simulink model "PolyMIMOsystem"  (R2021b)
settings: Solver=VariableStepAuto  StartTime=0.0  StopTime=Nsim  RelTol=1e-3
values from neighbouring files (symbols this model uses):
  myseed = [7; 27]    [dataGen_WH.m]
  Ts = 1e-2    (= 0.01)    [dataGen_WH.m]
libraries: cstblocks x4
settings Model: Creator=Simone Pirrera  LastModifiedBy=simon

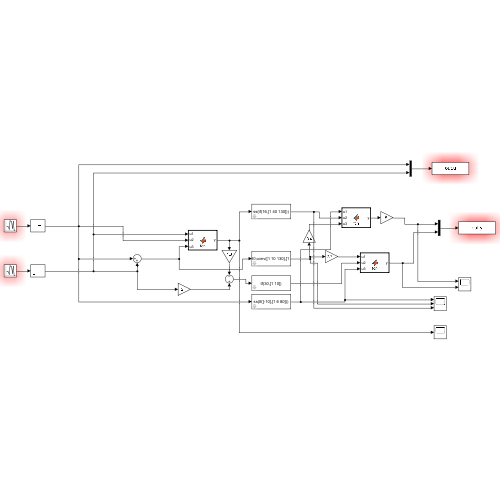
[thumbnail: Simulink's stored preview of the top-level diagram]
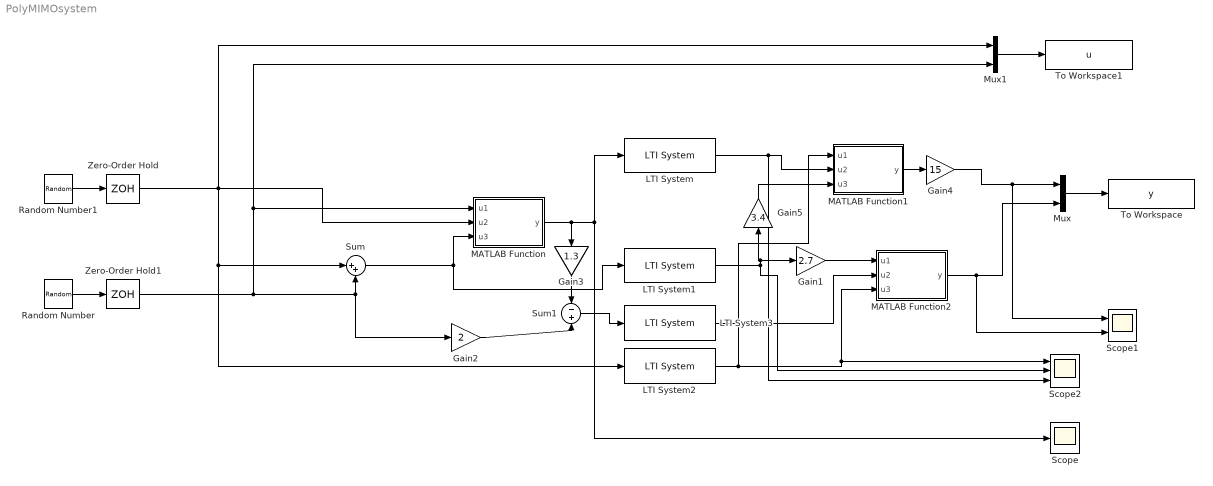
== system PolyMIMOsystem ==
  Gain1 : Gain  Gain=2.7
  Gain2 : Gain  Gain=2
  Gain3 : Gain  Gain=1.3
  Gain4 : Gain  Gain=15
  Gain5 : Gain  Gain=3.4
  LTI System : cstblocks/LTI System  sys=ss(tf(16,[1 40 130]))  IC=0.3*rand(2,1)
  LTI System1 : cstblocks/LTI System  sys=ss(tf(80,conv([1 10 130],[1 21])))  IC=0.1*randn(3,1)
  LTI System2 : cstblocks/LTI System  sys=ss(tf([-10],[1 6 80]))  IC=randn(2,1)
  LTI System3 : cstblocks/LTI System  sys=tf(30,[1 10])  IC=[]
  MATLAB Function : MATLAB Function  TreatAsAtomicUnit=on
  MATLAB Function1 : MATLAB Function  TreatAsAtomicUnit=on
  MATLAB Function2 : MATLAB Function  TreatAsAtomicUnit=on
  Mux : Mux  Inputs=2
  Mux1 : Mux  Inputs=2
  Random Number : RandomNumber  Seed=myseed(2)  SampleTime=Ts*100
  Random Number1 : RandomNumber  Seed=myseed(1)  SampleTime=Ts*100
  Scope : Scope
  Scope1 : Scope  NumInputPorts=2
  Scope2 : Scope  NumInputPorts=3
  Sum : Sum  Inputs=|++
  Sum1 : Sum  Inputs=-+
  To Workspace : ToWorkspace  VariableName=y  SaveFormat=Timeseries  SampleTime=Ts
  To Workspace1 : ToWorkspace  VariableName=u  SaveFormat=Timeseries  SampleTime=Ts
  Zero-Order Hold : ZeroOrderHold  SampleTime=-1
  Zero-Order Hold1 : ZeroOrderHold  SampleTime=-1
  wires:
  Random Number1/1 -> Zero-Order Hold/1
  Random Number/1 -> Zero-Order Hold1/1
  Mux/1 -> To Workspace/1
  Mux1/1 -> To Workspace1/1
  Zero-Order Hold1/1 -> Gain2/1, Sum/2, MATLAB Function/1(u1), Mux1/2
  MATLAB Function/1(y) -> Scope/1, LTI System/1, Gain3/1
  MATLAB Function1/1(y) -> Gain4/1
  Zero-Order Hold/1 -> LTI System2/1, Sum/1, MATLAB Function/2(u2), Mux1/1
  LTI System/1 -> Scope2/3, MATLAB Function1/2(u2)
  Sum/1 -> LTI System1/1, MATLAB Function/3(u3)
  LTI System1/1 -> Scope2/2, Gain5/1, Gain1/1
  LTI System3/1 -> MATLAB Function2/2(u2)
  Sum1/1 -> LTI System3/1
  MATLAB Function2/1(y) -> Scope1/2, Mux/2
  Gain1/1 -> MATLAB Function2/1(u1)
  Gain2/1 -> Sum1/2
  Gain3/1 -> Sum1/1
  LTI System2/1 -> MATLAB Function1/1(u1), Scope2/1, MATLAB Function2/3(u3)
  Gain4/1 -> Scope1/1, Mux/1
  Gain5/1 -> MATLAB Function1/3(u3)

== matlab function PolyMIMOsystem/MATLAB Function ==
  data: u1 input; y output; u2 input; u3 input
function y = fcn(u1,u2,u3)

y = 0.2*u1*u2 - u3 - 0.04*(u1^2)*u3;

== matlab function PolyMIMOsystem/MATLAB Function2 ==
  data: u1 input; y output; u2 input; u3 input
function y = fcn(u1,u2,u3)

y = u1*u2 - 0.1*u3*u1^2;

== matlab function PolyMIMOsystem/MATLAB Function1 ==
  data: u1 input; y output; u2 input; u3 input
function y = fcn(u1,u2,u3)

y = 0.5*u1*u2 - u3 + 0.02*u1^2*u3 - 0.6*u2^3;
